simulink model "EulerPIDJoint_Copy"  (Simulink 7.6)
settings: Solver=ode3  StartTime=0.0  StopTime=8  FixedStep=Ts  RelTol=1e-3
InitFcn:
  | eval('Config');
  | eval('RobotCtlCfg');
values from neighbouring files (symbols this model uses):
  a2 = 0    [Config.m]    (also in CtrPlatformCfg.m)
  a3 = 0    [Config.m]    (also in CtrPlatformCfg.m)
  a4 = 0    [Config.m]    (also in CtrPlatformCfg.m)
  a5 = 90    [Config.m]    (also in CtrPlatformCfg.m)
  a6 = 0    [Config.m]    (also in CtrPlatformCfg.m)
  Cen_EU = Cen    [DynEulerTest.m]
  DH_EU = [266     300     0       0       1016     0      174 ... (first row only)    [DynEulerTest.m]
  freq = tvel/radius    (= 1)    [Config.m]    (also in CtrPlatformCfg.m)
  Ft_EU = [0;0;0;0;0;0]    [DynEulerTest.m]
  Gravity = 9.8    [Config.m]    (also in CtrPlatformCfg.m)
  Ie_EU = [Ie1;Ie2;Ie3;Ie4;Ie5;Ie6]    [DynEulerTest.m]
  in1 = [5.2954 -0.2565 -0.6366;-0.2565 4.7000 0.2830;-0.6366 0.2829 5.8635]    [Config.m]    (also in CtrPlatformCfg.m; DynEulerTest.m; EfDynCAD.m = [0.54  -0.01 0.23)
  in2 = [5.8840 0.0072 0.0135;0.0072 6.0178 -0.1907;0.0135 -0.1907 0.3374]    [Config.m]    (also in CtrPlatformCfg.m; DynEulerTest.m; EfDynCAD.m = (R_x*R_z)*in2*(R_x*R_z)')
  in3 = [1.8201 -0.2274 -0.3112;-0.2274 2.2537 -0.1441;-0.3112 -0.1441 1.9485]    [Config.m]    (also in CtrPlatformCfg.m; DynEulerTest.m; EfDynCAD.m = (R_x*R_z)*in3*(R_x*R_z)')
  in4 = [0.0607 -0.0922 0;-0.0922 1.4493 0;0 0 1.4620]    [Config.m]    (also in CtrPlatformCfg.m; DynEulerTest.m = [0.0607 -0.0922 0;-0.0922 1.4493 0;0 0,1.4620]; EfDynCAD.m = (R_y*Rz)*in4*(R_y*Rz)')
  in5 = [0.0191 0.0032 0;0.0032 0.0228 0;0 0 0.0291]    [Config.m]    (also in CtrPlatformCfg.m; DynEulerTest.m; EfDynCAD.m = (R_x*R_y)*in5*(R_x*R_y)')
  in6 = [0.0012 0 0;0 0.0007 0;0 0 0.0007]    [Config.m]    (also in CtrPlatformCfg.m; DynEulerTest.m; EfDynCAD.m = (R_y*Rz)*in6*(R_y*Rz)')
  init_Endx = gd_init(1,4)    [Config.m]    (also in CtrPlatformCfg.m)
  init_Endy = gd_init(2,4)    [Config.m]    (also in CtrPlatformCfg.m)
  init_Endz = gd_init(3,4)    [Config.m]    (also in CtrPlatformCfg.m)
  init_Rot = gd_init(1:3,1:3)    [Config.m]    (also in CtrPlatformCfg.m)
  L = [l1 l2 l3 l4 l5 l6 l7 l8 l9]    [Config.m]    (also in CtrPlatformCfg.m)
  ma1 = 170.31    [Config.m]    (also in CtrPlatformCfg.m; DynEulerTest.m; EfDynCAD.m = 77.75)
  ma2 = 63.74    [Config.m]    (also in CtrPlatformCfg.m; DynEulerTest.m; EfDynCAD.m = 32.31)
  ma3 = 98.98    [Config.m]    (also in CtrPlatformCfg.m; DynEulerTest.m; EfDynCAD.m = 18.61)
  ma4 = 24.46    [Config.m]    (also in CtrPlatformCfg.m; DynEulerTest.m; EfDynCAD.m = 15.65)
  ma5 = 5.24    [Config.m]    (also in CtrPlatformCfg.m; DynEulerTest.m; EfDynCAD.m = 3.32)
  ma6 = 0.6    [Config.m]    (also in CtrPlatformCfg.m; DynEulerTest.m; EfDynCAD.m)
  Ma_EU = Ma    [DynEulerTest.m]
  Rad2Line = Gear*EncRes/(2*pi)    [Config.m]    (also in CtrPlatformCfg.m)
  Ts = 1/FrHz    (= 0.00025)    [Config.m]    (also in CtrPlatformCfg.m)
  tvel = 120    [Config.m]    (also in CtrPlatformCfg.m)
undefined symbols (not defined in the file or in its folder): a1, DiscIntNeverNeededParam, jointAugKp, jointAugKv, PRBSGain, PRBSOffset, PRBSTimeLength, PulseFrq, PulseGain, RobotAxis, SineFrq, SineGain, V2T
libraries: simulink x58, mblibv1 x41, powerlib_extras x7
(part 2 of 5)

== system EulerPIDJoint_Copy/Fanuc/ BodySensor 5 ==
  Avx : Scope
      settings: TimeRange=3  YMin=-150  YMax=125  SaveName=ScopeData62
  Avy : Scope
      settings: TimeRange=3  YMin=-150  YMax=125  SaveName=ScopeData63
  Avz : Scope
      settings: TimeRange=3  YMin=-150  YMax=125  SaveName=ScopeData64
  Awx : Scope
      settings: TimeRange=3  YMin=-150  YMax=125  SaveName=ScopeData65
  Awy : Scope
      settings: TimeRange=3  YMin=-150  YMax=125  SaveName=ScopeData66
  Awz : Scope
      settings: TimeRange=3  YMin=-150  YMax=125  SaveName=ScopeData67
  "Body Sensor " : mblibv1/Sensors &  Actuators/Body Sensor  DialogController=MECH.DynMechDlgSource  SystemSampleTime=-1  UpdateFromCAD=off  PhysicalDomain=Mechanical  PortType=blob  Muxed=on  Pose=off  Angle=on  AngleUnits=deg  ArcVelocity=on  ArcVelocityUnits=deg/s  ArcAcceleration=on  ArcAccelerationUnits=deg/s^2  CoordPosition=off  CoordPositionUnits=mm  Velocity=on  VelocityUnits=mm/s  Acceleration=on  AccelerationUnits=mm/s^2  Quaternion=on  QuaternionDT=off  QuaternionDDT=off  QuaternionUnits=off  OutputVector=[1]  ActiveIO=on  Width=12  DialogClass=MechanicalSensorBlock  ReferenceFrame=Local (Body CS)
  Demux5 : Demux  Outputs=12
  Vx : Scope
      settings: TimeRange=3  YMin=-150  YMax=125  SaveName=ScopeData55
  Vy : Scope
      settings: TimeRange=3  YMin=-150  YMax=125  SaveName=ScopeData57
  Vz : Scope
      settings: TimeRange=3  YMin=-150  YMax=125  SaveName=ScopeData58
  wx : Scope
      settings: TimeRange=3  YMin=-150  YMax=125  SaveName=ScopeData59
  wy : Scope
      settings: TimeRange=3  YMin=-150  YMax=125  SaveName=ScopeData60
  wz : Scope
      settings: TimeRange=3  YMin=-150  YMax=125  SaveName=ScopeData61
  In : PMIOPort  Port=1  Side=Left
  Out : Outport
  wires:
  Demux5/12 -> Awz/1
  Demux5/11 -> Awy/1
  Demux5/10 -> Awx/1
  Demux5/9 -> Avz/1
  Demux5/8 -> Avy/1
  Demux5/7 -> Avx/1
  Demux5/6 -> wz/1
  Demux5/5 -> wy/1
  Demux5/4 -> wx/1
  Demux5/3 -> Vz/1
  Demux5/2 -> Vy/1
  Demux5/1 -> Vx/1
  "Body Sensor "/1 -> Demux5/1, Out/1
  connections:
  In/RConn1 -- "Body Sensor "/LConn1

== system EulerPIDJoint_Copy/Fanuc/ BodySensor 6 ==
  Avx : Scope
      settings: TimeRange=3  YMin=-150  YMax=125  SaveName=ScopeData62
  Avy : Scope
      settings: TimeRange=3  YMin=-150  YMax=125  SaveName=ScopeData63
  Avz : Scope
      settings: TimeRange=3  YMin=-150  YMax=125  SaveName=ScopeData64
  Awx : Scope
      settings: TimeRange=3  YMin=-150  YMax=125  SaveName=ScopeData65
  Awy : Scope
      settings: TimeRange=3  YMin=-150  YMax=125  SaveName=ScopeData66
  Awz : Scope
      settings: TimeRange=3  YMin=-150  YMax=125  SaveName=ScopeData67
  "Body Sensor " : mblibv1/Sensors &  Actuators/Body Sensor  DialogController=MECH.DynMechDlgSource  SystemSampleTime=-1  UpdateFromCAD=off  PhysicalDomain=Mechanical  PortType=blob  Muxed=on  Pose=off  Angle=on  AngleUnits=deg  ArcVelocity=on  ArcVelocityUnits=deg/s  ArcAcceleration=on  ArcAccelerationUnits=deg/s^2  CoordPosition=off  CoordPositionUnits=mm  Velocity=on  VelocityUnits=mm/s  Acceleration=on  AccelerationUnits=mm/s^2  Quaternion=on  QuaternionDT=off  QuaternionDDT=off  QuaternionUnits=off  OutputVector=[1]  ActiveIO=on  Width=12  DialogClass=MechanicalSensorBlock  ReferenceFrame=Local (Body CS)
  Demux5 : Demux  Outputs=12
  Vx : Scope
      settings: TimeRange=3  YMin=-150  YMax=125  SaveName=ScopeData55
  Vy : Scope
      settings: TimeRange=3  YMin=-150  YMax=125  SaveName=ScopeData57
  Vz : Scope
      settings: TimeRange=3  YMin=-150  YMax=125  SaveName=ScopeData58
  wx : Scope
      settings: TimeRange=3  YMin=-150  YMax=125  SaveName=ScopeData59
  wy : Scope
      settings: TimeRange=3  YMin=-150  YMax=125  SaveName=ScopeData60
  wz : Scope
      settings: TimeRange=3  YMin=-150  YMax=125  SaveName=ScopeData61
  In : PMIOPort  Port=1  Side=Left
  Out : Outport
  wires:
  "Body Sensor "/1 -> Out/1, Demux5/1
  Demux5/1 -> Vx/1
  Demux5/2 -> Vy/1
  Demux5/3 -> Vz/1
  Demux5/4 -> wx/1
  Demux5/5 -> wy/1
  Demux5/6 -> wz/1
  Demux5/7 -> Avx/1
  Demux5/8 -> Avy/1
  Demux5/9 -> Avz/1
  Demux5/10 -> Awx/1
  Demux5/11 -> Awy/1
  Demux5/12 -> Awz/1
  connections:
  In/RConn1 -- "Body Sensor "/LConn1

== system EulerPIDJoint_Copy/Fanuc/ EndSensor ==
  Avx : Scope
      settings: TimeRange=3  YMin=-150  YMax=125  SaveName=ScopeData62
  Avy : Scope
      settings: TimeRange=3  YMin=-150  YMax=125  SaveName=ScopeData63
  Avz : Scope
      settings: TimeRange=3  YMin=-150  YMax=125  SaveName=ScopeData64
  Awx : Scope
      settings: TimeRange=3  YMin=-150  YMax=125  SaveName=ScopeData65
  Awy : Scope
      settings: TimeRange=3  YMin=-150  YMax=125  SaveName=ScopeData66
  Awz : Scope
      settings: TimeRange=3  YMin=-150  YMax=125  SaveName=ScopeData67
  "Body Sensor " : mblibv1/Sensors &  Actuators/Body Sensor  DialogController=MECH.DynMechDlgSource  SystemSampleTime=-1  UpdateFromCAD=off  PhysicalDomain=Mechanical  PortType=blob  Muxed=on  Pose=off  Angle=on  AngleUnits=deg  ArcVelocity=on  ArcVelocityUnits=deg/s  ArcAcceleration=on  ArcAccelerationUnits=deg/s^2  CoordPosition=on  CoordPositionUnits=mm  Velocity=on  VelocityUnits=mm/s  Acceleration=on  AccelerationUnits=mm/s^2  Quaternion=on  QuaternionDT=off  QuaternionDDT=off  QuaternionUnits=off  OutputVector=[1]  ActiveIO=on  Width=15  DialogClass=MechanicalSensorBlock  ReferenceFrame=Absolute (World)
  Demux5 : Demux  Outputs=15
  EndX : ToWorkspace  VariableName=EndX  SampleTime=-1  SaveFormat=Structure
  EndY : ToWorkspace  VariableName=EndY  SampleTime=-1  SaveFormat=Structure
  EndZ : ToWorkspace  VariableName=EndZ  SampleTime=-1  SaveFormat=Structure
  Vx : Scope
      settings: TimeRange=3  YMin=-150  YMax=125  SaveName=ScopeData55
  Vy : Scope
      settings: TimeRange=3  YMin=-150  YMax=125  SaveName=ScopeData57
  Vz : Scope
      settings: TimeRange=3  YMin=-150  YMax=125  SaveName=ScopeData58
  X : Scope
      settings: TimeRange=3  YMin=-150  YMax=125  SaveName=ScopeData36
  Y : Scope
      settings: TimeRange=3  YMin=-150  YMax=125  SaveName=ScopeData37
  Z : Scope
      settings: TimeRange=3  YMin=-150  YMax=125  SaveName=ScopeData38
  wx : Scope
      settings: TimeRange=3  YMin=-150  YMax=125  SaveName=ScopeData59
  wy : Scope
      settings: TimeRange=3  YMin=-150  YMax=125  SaveName=ScopeData60
  wz : Scope
      settings: TimeRange=3  YMin=-150  YMax=125  SaveName=ScopeData61
  In : PMIOPort  Port=1  Side=Left
  Out : Outport
  wires:
  "Body Sensor "/1 -> Demux5/1, Out/1
  Demux5/4 -> Vx/1
  Demux5/5 -> Vy/1
  Demux5/6 -> Vz/1
  Demux5/7 -> wx/1
  Demux5/8 -> wy/1
  Demux5/9 -> wz/1
  Demux5/10 -> Avx/1
  Demux5/11 -> Avy/1
  Demux5/12 -> Avz/1
  Demux5/13 -> Awx/1
  Demux5/14 -> Awy/1
  Demux5/15 -> Awz/1
  Demux5/1 -> EndX/1, X/1
  Demux5/2 -> EndY/1, Y/1
  Demux5/3 -> EndZ/1, Z/1
  connections:
  In/RConn1 -- "Body Sensor "/LConn1

== system EulerPIDJoint_Copy/Fanuc/JointSensor1 ==
  Angle Acceleration : Scope
      settings: SaveName=ScopeData32
  Angle Velocity : Scope
      settings: SaveName=ScopeData31
  Anlge : Scope
      settings: SaveName=ScopeData30
  Computed Torque : Scope
      settings: SaveName=ScopeData33
  Demux : Demux  Outputs=10
  Reaction Force : Scope  NumInputPorts=3
      settings: YMin=-5~-5~-5  YMax=5~5~5  SaveName=ScopeData12
  Reaction Torque : Scope  NumInputPorts=3
      settings: YMin=-5~-5~-5  YMax=5~5~5  SaveName=ScopeData34
  Sensor1 : mblibv1/Sensors &  Actuators/Joint Sensor  DialogController=MECH.DynMechDlgSource  SystemSampleTime=-1  UpdateFromCAD=off  PhysicalDomain=Mechanical  PortType=blob  Muxed=on  Pose=off  Angle=on  AngleUnits=deg  ArcVelocity=on  ArcVelocityUnits=deg/s  ArcAcceleration=on  ArcAccelerationUnits=deg/s^2  CoordPosition=on  CoordPositionUnits=m  Velocity=off  VelocityUnits=m/s  Acceleration=off  AccelerationUnits=m/s^2  Quaternion=on  QuaternionDT=off  QuaternionDDT=off  QuaternionUnits=off  OutputVector=[1]  ActiveIO=on  Width=10  DialogClass=MechanicalSensorBlock  Primitive=R1  Force=off  ForceUnits=N  Torque=on  TorqueUnits=N*m  ReferenceFrame=Absolute (World)  ReactionSensedSide=Follower  ReactionReferenceFrame=Absolute (World)  ReactionForce=on  ReactionForceUnits=N  ReactionMoment=on  ReactionMomentUnits=N*m
  In : PMIOPort  Port=1  Side=Left
  Out : Outport
  wires:
  Sensor1/1 -> Demux/1, Out/1
  Demux/2 -> Angle Velocity/1
  Demux/1 -> Anlge/1
  Demux/3 -> Angle Acceleration/1
  Demux/4 -> Computed Torque/1
  Demux/5 -> Reaction Torque/1
  Demux/6 -> Reaction Torque/2
  Demux/7 -> Reaction Torque/3
  Demux/8 -> Reaction Force/1
  Demux/9 -> Reaction Force/2
  Demux/10 -> Reaction Force/3
  connections:
  In/RConn1 -- Sensor1/LConn1

== system EulerPIDJoint_Copy/Fanuc/JointSensor2 ==
  Angle Acceleration : Scope
      settings: SaveName=ScopeData32
  Angle Velocity : Scope
      settings: SaveName=ScopeData31
  Anlge : Scope
      settings: SaveName=ScopeData30
  Computed Torque : Scope
      settings: SaveName=ScopeData33
  Demux : Demux  Outputs=10
  Reaction Force : Scope  NumInputPorts=3
      settings: YMin=-5~-5~-5  YMax=5~5~5  SaveName=ScopeData12
  Reaction Torque : Scope  NumInputPorts=3
      settings: YMin=-5~-5~-5  YMax=5~5~5  SaveName=ScopeData34
  Sensor1 : mblibv1/Sensors &  Actuators/Joint Sensor  DialogController=MECH.DynMechDlgSource  SystemSampleTime=-1  UpdateFromCAD=off  PhysicalDomain=Mechanical  PortType=blob  Muxed=on  Pose=off  Angle=on  AngleUnits=deg  ArcVelocity=on  ArcVelocityUnits=deg/s  ArcAcceleration=on  ArcAccelerationUnits=deg/s^2  CoordPosition=on  CoordPositionUnits=m  Velocity=off  VelocityUnits=m/s  Acceleration=off  AccelerationUnits=m/s^2  Quaternion=on  QuaternionDT=off  QuaternionDDT=off  QuaternionUnits=off  OutputVector=[1]  ActiveIO=on  Width=10  DialogClass=MechanicalSensorBlock  Primitive=R1  Force=off  ForceUnits=N  Torque=on  TorqueUnits=N*m  ReferenceFrame=Absolute (World)  ReactionSensedSide=Follower  ReactionReferenceFrame=Absolute (World)  ReactionForce=on  ReactionForceUnits=N  ReactionMoment=on  ReactionMomentUnits=N*m
  In : PMIOPort  Port=1  Side=Left
  Out : Outport
  wires:
  Demux/10 -> Reaction Force/3
  Demux/9 -> Reaction Force/2
  Demux/8 -> Reaction Force/1
  Demux/7 -> Reaction Torque/3
  Demux/6 -> Reaction Torque/2
  Demux/5 -> Reaction Torque/1
  Demux/4 -> Computed Torque/1
  Demux/3 -> Angle Acceleration/1
  Demux/1 -> Anlge/1
  Demux/2 -> Angle Velocity/1
  Sensor1/1 -> Out/1, Demux/1
  connections:
  In/RConn1 -- Sensor1/LConn1

== system EulerPIDJoint_Copy/Fanuc/JointSensor3 ==
  Angle Acceleration : Scope
      settings: SaveName=ScopeData32
  Angle Velocity : Scope
      settings: SaveName=ScopeData31
  Anlge : Scope
      settings: SaveName=ScopeData30
  Computed Torque : Scope
      settings: SaveName=ScopeData33
  Demux : Demux  Outputs=10
  Reaction Force : Scope  NumInputPorts=3
      settings: YMin=-5~-5~-5  YMax=5~5~5  SaveName=ScopeData12
  Reaction Torque : Scope  NumInputPorts=3
      settings: YMin=-5~-5~-5  YMax=5~5~5  SaveName=ScopeData34
  Sensor1 : mblibv1/Sensors &  Actuators/Joint Sensor  DialogController=MECH.DynMechDlgSource  SystemSampleTime=-1  UpdateFromCAD=off  PhysicalDomain=Mechanical  PortType=blob  Muxed=on  Pose=off  Angle=on  AngleUnits=deg  ArcVelocity=on  ArcVelocityUnits=deg/s  ArcAcceleration=on  ArcAccelerationUnits=deg/s^2  CoordPosition=on  CoordPositionUnits=m  Velocity=off  VelocityUnits=m/s  Acceleration=off  AccelerationUnits=m/s^2  Quaternion=on  QuaternionDT=off  QuaternionDDT=off  QuaternionUnits=off  OutputVector=[1]  ActiveIO=on  Width=10  DialogClass=MechanicalSensorBlock  Primitive=R1  Force=off  ForceUnits=N  Torque=on  TorqueUnits=N*m  ReferenceFrame=Absolute (World)  ReactionSensedSide=Follower  ReactionReferenceFrame=Absolute (World)  ReactionForce=on  ReactionForceUnits=N  ReactionMoment=on  ReactionMomentUnits=N*m
  In : PMIOPort  Port=1  Side=Left
  Out : Outport
  wires:
  Sensor1/1 -> Demux/1, Out/1
  Demux/2 -> Angle Velocity/1
  Demux/1 -> Anlge/1
  Demux/3 -> Angle Acceleration/1
  Demux/4 -> Computed Torque/1
  Demux/5 -> Reaction Torque/1
  Demux/6 -> Reaction Torque/2
  Demux/7 -> Reaction Torque/3
  Demux/8 -> Reaction Force/1
  Demux/9 -> Reaction Force/2
  Demux/10 -> Reaction Force/3
  connections:
  In/RConn1 -- Sensor1/LConn1

== system EulerPIDJoint_Copy/Fanuc/JointSensor4 ==
  Angle Acceleration : Scope
      settings: SaveName=ScopeData32
  Angle Velocity : Scope
      settings: SaveName=ScopeData31
  Anlge : Scope
      settings: SaveName=ScopeData30
  Computed Torque : Scope
      settings: SaveName=ScopeData33
  Demux : Demux  Outputs=10
  Reaction Force : Scope  NumInputPorts=3
      settings: YMin=-5~-5~-5  YMax=5~5~5  SaveName=ScopeData12
  Reaction Torque : Scope  NumInputPorts=3
      settings: YMin=-5~-5~-5  YMax=5~5~5  SaveName=ScopeData34
  Sensor1 : mblibv1/Sensors &  Actuators/Joint Sensor  DialogController=MECH.DynMechDlgSource  SystemSampleTime=-1  UpdateFromCAD=off  PhysicalDomain=Mechanical  PortType=blob  Muxed=on  Pose=off  Angle=on  AngleUnits=deg  ArcVelocity=on  ArcVelocityUnits=deg/s  ArcAcceleration=on  ArcAccelerationUnits=deg/s^2  CoordPosition=on  CoordPositionUnits=m  Velocity=off  VelocityUnits=m/s  Acceleration=off  AccelerationUnits=m/s^2  Quaternion=on  QuaternionDT=off  QuaternionDDT=off  QuaternionUnits=off  OutputVector=[1]  ActiveIO=on  Width=10  DialogClass=MechanicalSensorBlock  Primitive=R1  Force=off  ForceUnits=N  Torque=on  TorqueUnits=N*m  ReferenceFrame=Absolute (World)  ReactionSensedSide=Follower  ReactionReferenceFrame=Absolute (World)  ReactionForce=on  ReactionForceUnits=N  ReactionMoment=on  ReactionMomentUnits=N*m
  In : PMIOPort  Port=1  Side=Left
  Out : Outport
  wires:
  Demux/10 -> Reaction Force/3
  Demux/9 -> Reaction Force/2
  Demux/8 -> Reaction Force/1
  Demux/7 -> Reaction Torque/3
  Demux/6 -> Reaction Torque/2
  Demux/5 -> Reaction Torque/1
  Demux/4 -> Computed Torque/1
  Demux/3 -> Angle Acceleration/1
  Demux/1 -> Anlge/1
  Demux/2 -> Angle Velocity/1
  Sensor1/1 -> Out/1, Demux/1
  connections:
  In/RConn1 -- Sensor1/LConn1

== system EulerPIDJoint_Copy/Fanuc/JointSensor5 ==
  Angle Acceleration : Scope
      settings: SaveName=ScopeData32
  Angle Velocity : Scope
      settings: SaveName=ScopeData31
  Anlge : Scope
      settings: SaveName=ScopeData30
  Computed Torque : Scope
      settings: SaveName=ScopeData33
  Demux : Demux  Outputs=10
  Reaction Force : Scope  NumInputPorts=3
      settings: YMin=-5~-5~-5  YMax=5~5~5  SaveName=ScopeData12
  Reaction Torque : Scope  NumInputPorts=3
      settings: YMin=-5~-5~-5  YMax=5~5~5  SaveName=ScopeData34
  Sensor1 : mblibv1/Sensors &  Actuators/Joint Sensor  DialogController=MECH.DynMechDlgSource  SystemSampleTime=-1  UpdateFromCAD=off  PhysicalDomain=Mechanical  PortType=blob  Muxed=on  Pose=off  Angle=on  AngleUnits=deg  ArcVelocity=on  ArcVelocityUnits=deg/s  ArcAcceleration=on  ArcAccelerationUnits=deg/s^2  CoordPosition=on  CoordPositionUnits=m  Velocity=off  VelocityUnits=m/s  Acceleration=off  AccelerationUnits=m/s^2  Quaternion=on  QuaternionDT=off  QuaternionDDT=off  QuaternionUnits=off  OutputVector=[1]  ActiveIO=on  Width=10  DialogClass=MechanicalSensorBlock  Primitive=R1  Force=off  ForceUnits=N  Torque=on  TorqueUnits=N*m  ReferenceFrame=Absolute (World)  ReactionSensedSide=Follower  ReactionReferenceFrame=Absolute (World)  ReactionForce=on  ReactionForceUnits=N  ReactionMoment=on  ReactionMomentUnits=N*m
  In : PMIOPort  Port=1  Side=Left
  Out : Outport
  wires:
  Sensor1/1 -> Demux/1, Out/1
  Demux/2 -> Angle Velocity/1
  Demux/1 -> Anlge/1
  Demux/3 -> Angle Acceleration/1
  Demux/4 -> Computed Torque/1
  Demux/5 -> Reaction Torque/1
  Demux/6 -> Reaction Torque/2
  Demux/7 -> Reaction Torque/3
  Demux/8 -> Reaction Force/1
  Demux/9 -> Reaction Force/2
  Demux/10 -> Reaction Force/3
  connections:
  In/RConn1 -- Sensor1/LConn1

== system EulerPIDJoint_Copy/Fanuc/JointSensor6 ==
  Angle Acceleration : Scope
      settings: SaveName=ScopeData32
  Angle Velocity : Scope
      settings: SaveName=ScopeData31
  Anlge : Scope
      settings: SaveName=ScopeData30
  Computed Torque : Scope
      settings: SaveName=ScopeData33
  Demux : Demux  Outputs=10
  Reaction Force : Scope  NumInputPorts=3
      settings: YMin=-5~-5~-5  YMax=5~5~5  SaveName=ScopeData12
  Reaction Torque : Scope  NumInputPorts=3
      settings: YMin=-5~-5~-5  YMax=5~5~5  SaveName=ScopeData34
  Sensor1 : mblibv1/Sensors &  Actuators/Joint Sensor  DialogController=MECH.DynMechDlgSource  SystemSampleTime=-1  UpdateFromCAD=off  PhysicalDomain=Mechanical  PortType=blob  Muxed=on  Pose=off  Angle=on  AngleUnits=deg  ArcVelocity=on  ArcVelocityUnits=deg/s  ArcAcceleration=on  ArcAccelerationUnits=deg/s^2  CoordPosition=on  CoordPositionUnits=m  Velocity=off  VelocityUnits=m/s  Acceleration=off  AccelerationUnits=m/s^2  Quaternion=on  QuaternionDT=off  QuaternionDDT=off  QuaternionUnits=off  OutputVector=[1]  ActiveIO=on  Width=10  DialogClass=MechanicalSensorBlock  Primitive=R1  Force=off  ForceUnits=N  Torque=on  TorqueUnits=N*m  ReferenceFrame=Absolute (World)  ReactionSensedSide=Follower  ReactionReferenceFrame=Absolute (World)  ReactionForce=on  ReactionForceUnits=N  ReactionMoment=on  ReactionMomentUnits=N*m
  In : PMIOPort  Port=1  Side=Left
  Out : Outport
  wires:
  Demux/10 -> Reaction Force/3
  Demux/9 -> Reaction Force/2
  Demux/8 -> Reaction Force/1
  Demux/7 -> Reaction Torque/3
  Demux/6 -> Reaction Torque/2
  Demux/5 -> Reaction Torque/1
  Demux/4 -> Computed Torque/1
  Demux/3 -> Angle Acceleration/1
  Demux/1 -> Anlge/1
  Demux/2 -> Angle Velocity/1
  Sensor1/1 -> Out/1, Demux/1
  connections:
  In/RConn1 -- Sensor1/LConn1

== system EulerPIDJoint_Copy/Signal Re-group/Re-group ==
  JntVelAcc_R1 : Inport
  Torque_R1 : Inport  Port=2
  GeneralForce_R1 : Inport  Port=3
  JntVelAcc_R2 : Inport  Port=4
  Torque_R2 : Inport  Port=5
  GeneralForce_R2 : Inport  Port=6
  JntVelAcc_R3 : Inport  Port=7
  Torque_R3 : Inport  Port=8
  GeneralForce_R3 : Inport  Port=9
  JntVelAcc_R4 : Inport  Port=10
  Torque_R4 : Inport  Port=11
  GeneralForce_R4 : Inport  Port=12
  JntVelAcc_R5 : Inport  Port=13
  Torque_R5 : Inport  Port=14
  GeneralForce_R5 : Inport  Port=15
  JntVelAcc_R6 : Inport  Port=16
  Torque_R6 : Inport  Port=17
  GeneralForce_R6 : Inport  Port=18
  Mux : Mux  Inputs=6
  Mux1 : Mux  Inputs=6
  Mux2 : Mux  Inputs=6
  JntVelAcc : Outport
  Torque : Outport  Port=2
  GeneralForce : Outport  Port=3
  wires:
  JntVelAcc_R1/1 -> Mux/1
  JntVelAcc_R2/1 -> Mux/2
  JntVelAcc_R3/1 -> Mux/3
  JntVelAcc_R4/1 -> Mux/4
  JntVelAcc_R5/1 -> Mux/5
  JntVelAcc_R6/1 -> Mux/6
  Torque_R1/1 -> Mux1/1
  Torque_R2/1 -> Mux1/2
  Torque_R3/1 -> Mux1/3
  Torque_R4/1 -> Mux1/4
  Torque_R5/1 -> Mux1/5
  Torque_R6/1 -> Mux1/6
  GeneralForce_R1/1 -> Mux2/1
  GeneralForce_R2/1 -> Mux2/2
  GeneralForce_R3/1 -> Mux2/3
  GeneralForce_R4/1 -> Mux2/4
  GeneralForce_R5/1 -> Mux2/5
  GeneralForce_R6/1 -> Mux2/6
  Mux/1 -> JntVelAcc/1
  Mux1/1 -> Torque/1
  Mux2/1 -> GeneralForce/1

== system EulerPIDJoint_Copy/Signal Re-group/Re-group JntVelAcc ==
  JntVelAcc : Inport
  Demux2 : Demux  Outputs=18
  Mux : Mux  Inputs=6
  Mux1 : Mux  Inputs=6
  Mux2 : Mux  Inputs=6
  Mux3 : Mux  Inputs=3
  ReJntVelAcc : Outport
  wires:
  JntVelAcc/1 -> Demux2/1
  Demux2/1 -> Mux/1
  Demux2/2 -> Mux1/1
  Demux2/3 -> Mux2/1
  Demux2/4 -> Mux/2
  Demux2/5 -> Mux1/2
  Demux2/6 -> Mux2/2
  Demux2/7 -> Mux/3
  Demux2/8 -> Mux1/3
  Demux2/9 -> Mux2/3
  Demux2/10 -> Mux/4
  Demux2/11 -> Mux1/4
  Demux2/12 -> Mux2/4
  Demux2/13 -> Mux/5
  Demux2/14 -> Mux1/5
  Demux2/15 -> Mux2/5
  Demux2/16 -> Mux/6
  Demux2/17 -> Mux1/6
  Demux2/18 -> Mux2/6
  Mux/1 -> Mux3/1
  Mux1/1 -> Mux3/2
  Mux2/1 -> Mux3/3
  Mux3/1 -> ReJntVelAcc/1

== system EulerPIDJoint_Copy/Signal Re-group/Re-group_B ==
  In_B1 : Inport
  In_B2 : Inport  Port=2
  In_B3 : Inport  Port=3
  In_B4 : Inport  Port=4
  In_B5 : Inport  Port=5
  In_B6 : Inport  Port=6
  Demux{1..6} (6 alike) : Demux  Outputs=2
  Mux : Mux  Inputs=6
  Mux1 : Mux  Inputs=6
  GeneralVel : Outport
  GeneralAcc : Outport  Port=2
  wires:
  In_B1/1 -> Demux2/1
  In_B2/1 -> Demux1/1
  In_B3/1 -> Demux3/1
  In_B4/1 -> Demux4/1
  In_B5/1 -> Demux5/1
  In_B6/1 -> Demux6/1
  Demux2/1 -> Mux/1
  Demux1/1 -> Mux/2
  Demux3/1 -> Mux/3
  Demux4/1 -> Mux/4
  Demux5/1 -> Mux/5
  Demux6/1 -> Mux/6
  Demux2/2 -> Mux1/1
  Demux1/2 -> Mux1/2
  Demux3/2 -> Mux1/3
  Demux4/2 -> Mux1/4
  Demux5/2 -> Mux1/5
  Demux6/2 -> Mux1/6
  Mux1/1 -> GeneralAcc/1
  Mux/1 -> GeneralVel/1

== system EulerPIDJoint_Copy/Signal Re-group/Re-group_R1 ==
  In_R1 : Inport
  Demux2 : Demux  Outputs=10
  Mux : Mux  Inputs=3
  Mux1 : Mux  Inputs=3
  Mux2 : Mux  Inputs=3
  Mux3 : Mux  Inputs=2
  JntVelAcc_R1 : Outport
  Torque_R1 : Outport  Port=2
  GeneralForce_R1 : Outport  Port=3
  wires:
  In_R1/1 -> Demux2/1
  Demux2/1 -> Mux/1
  Demux2/2 -> Mux/2
  Demux2/3 -> Mux/3
  Demux2/4 -> Torque_R1/1
  Demux2/5 -> Mux1/1
  Demux2/6 -> Mux1/2
  Demux2/7 -> Mux1/3
  Demux2/8 -> Mux2/1
  Demux2/9 -> Mux2/2
  Demux2/10 -> Mux2/3
  Mux1/1 -> Mux3/2
  Mux2/1 -> Mux3/1
  Mux/1 -> JntVelAcc_R1/1
  Mux3/1 -> GeneralForce_R1/1

== system EulerPIDJoint_Copy/Signal Re-group/Re-group_R2 ==
  In_R2 : Inport
  Demux2 : Demux  Outputs=10
  Mux : Mux  Inputs=3
  Mux1 : Mux  Inputs=3
  Mux2 : Mux  Inputs=3
  Mux3 : Mux  Inputs=2
  JntVelAcc_R2 : Outport
  Torque_R2 : Outport  Port=2
  GeneralForce_R2 : Outport  Port=3
  wires:
  Mux3/1 -> GeneralForce_R2/1
  Mux/1 -> JntVelAcc_R2/1
  Mux2/1 -> Mux3/1
  Mux1/1 -> Mux3/2
  Demux2/10 -> Mux2/3
  Demux2/9 -> Mux2/2
  Demux2/8 -> Mux2/1
  Demux2/7 -> Mux1/3
  Demux2/6 -> Mux1/2
  Demux2/5 -> Mux1/1
  Demux2/4 -> Torque_R2/1
  Demux2/3 -> Mux/3
  Demux2/2 -> Mux/2
  Demux2/1 -> Mux/1
  In_R2/1 -> Demux2/1

== system EulerPIDJoint_Copy/Signal Re-group/Re-group_R3 ==
  In_R3 : Inport
  Demux2 : Demux  Outputs=10
  Mux : Mux  Inputs=3
  Mux1 : Mux  Inputs=3
  Mux2 : Mux  Inputs=3
  Mux3 : Mux  Inputs=2
  JntVelAcc_R3 : Outport
  Torque_R3 : Outport  Port=2
  GeneralForce_R3 : Outport  Port=3
  wires:
  In_R3/1 -> Demux2/1
  Demux2/1 -> Mux/1
  Demux2/2 -> Mux/2
  Demux2/3 -> Mux/3
  Demux2/4 -> Torque_R3/1
  Demux2/5 -> Mux1/1
  Demux2/6 -> Mux1/2
  Demux2/7 -> Mux1/3
  Demux2/8 -> Mux2/1
  Demux2/9 -> Mux2/2
  Demux2/10 -> Mux2/3
  Mux1/1 -> Mux3/2
  Mux2/1 -> Mux3/1
  Mux/1 -> JntVelAcc_R3/1
  Mux3/1 -> GeneralForce_R3/1

== system EulerPIDJoint_Copy/Signal Re-group/Re-group_R4 ==
  In_R4 : Inport
  Demux2 : Demux  Outputs=10
  Mux : Mux  Inputs=3
  Mux1 : Mux  Inputs=3
  Mux2 : Mux  Inputs=3
  Mux3 : Mux  Inputs=2
  JntVelAcc_R4 : Outport
  Torque_R4 : Outport  Port=2
  GeneralForce_R4 : Outport  Port=3
  wires:
  Mux3/1 -> GeneralForce_R4/1
  Mux/1 -> JntVelAcc_R4/1
  Mux2/1 -> Mux3/1
  Mux1/1 -> Mux3/2
  Demux2/10 -> Mux2/3
  Demux2/9 -> Mux2/2
  Demux2/8 -> Mux2/1
  Demux2/7 -> Mux1/3
  Demux2/6 -> Mux1/2
  Demux2/5 -> Mux1/1
  Demux2/4 -> Torque_R4/1
  Demux2/3 -> Mux/3
  Demux2/2 -> Mux/2
  Demux2/1 -> Mux/1
  In_R4/1 -> Demux2/1

== system EulerPIDJoint_Copy/Signal Re-group/Re-group_R5 ==
  In_R5 : Inport
  Demux2 : Demux  Outputs=10
  Mux : Mux  Inputs=3
  Mux1 : Mux  Inputs=3
  Mux2 : Mux  Inputs=3
  Mux3 : Mux  Inputs=2
  JntVelAcc_R5 : Outport
  Torque_R5 : Outport  Port=2
  GeneralForce_R5 : Outport  Port=3
  wires:
  In_R5/1 -> Demux2/1
  Demux2/1 -> Mux/1
  Demux2/2 -> Mux/2
  Demux2/3 -> Mux/3
  Demux2/4 -> Torque_R5/1
  Demux2/5 -> Mux1/1
  Demux2/6 -> Mux1/2
  Demux2/7 -> Mux1/3
  Demux2/8 -> Mux2/1
  Demux2/9 -> Mux2/2
  Demux2/10 -> Mux2/3
  Mux1/1 -> Mux3/2
  Mux2/1 -> Mux3/1
  Mux/1 -> JntVelAcc_R5/1
  Mux3/1 -> GeneralForce_R5/1

== system EulerPIDJoint_Copy/Signal Re-group/Re-group_R6 ==
  In_R6 : Inport
  Demux2 : Demux  Outputs=10
  Mux : Mux  Inputs=3
  Mux1 : Mux  Inputs=3
  Mux2 : Mux  Inputs=3
  Mux3 : Mux  Inputs=2
  JntVelAcc_R6 : Outport
  Torque_R6 : Outport  Port=2
  GeneralForce_R6 : Outport  Port=3
  wires:
  Mux3/1 -> GeneralForce_R6/1
  Mux/1 -> JntVelAcc_R6/1
  Mux2/1 -> Mux3/1
  Mux1/1 -> Mux3/2
  Demux2/10 -> Mux2/3
  Demux2/9 -> Mux2/2
  Demux2/8 -> Mux2/1
  Demux2/7 -> Mux1/3
  Demux2/6 -> Mux1/2
  Demux2/5 -> Mux1/1
  Demux2/4 -> Torque_R6/1
  Demux2/3 -> Mux/3
  Demux2/2 -> Mux/2
  Demux2/1 -> Mux/1
  In_R6/1 -> Demux2/1

== system EulerPIDJoint_Copy/Trajectory Generator/Circle in Descartes Space ==
  Difference{,1..3} (4 alike) : simulink/Discrete/Difference  SystemSampleTime=-1  ICPrevInput=0.0  OutMin=[]  OutMax=[]  OutDataType=fixdt(1, 16)  OutScaling=2^-10  DoSatur=off
  Discrete-Time Integrator : DiscreteIntegrator  InitialCondition=init_Endx  SampleTime=Ts  ICPrevOutput=DiscIntNeverNeededParam  ICPrevScaledInput=DiscIntNeverNeededParam
  Discrete-Time Integrator1 : DiscreteIntegrator  InitialCondition=init_Endy  SampleTime=Ts  ICPrevOutput=DiscIntNeverNeededParam  ICPrevScaledInput=DiscIntNeverNeededParam
  Discrete-Time Integrator2 : DiscreteIntegrator  InitialCondition=init_Endz  SampleTime=Ts  ICPrevOutput=DiscIntNeverNeededParam  ICPrevScaledInput=DiscIntNeverNeededParam
  EndVelocity : Subsystem
  Inverse Kinematic : Stateflow chart  TreatAsAtomicUnit=on
  Jacobian : Stateflow chart  TreatAsAtomicUnit=on
  Mux{1..3,5..6} (5 alike) : Mux  Inputs=3
  Mux4 : Mux  Inputs=5
  Rad2Deg : Gain  Gain=180/pi
  "Re-group " : Subsystem
  Zero : Gain  Gain=0
  Zero1 : Gain  Gain=1/Ts
  Zero2 : Gain  Gain=1/Ts
  Ref_JJVVAA : Outport
  RefEnd : Outport  Port=2
  Ref_JVAJVA : Outport  Port=3
  wires:
  Discrete-Time Integrator/1 -> Mux2/1
  Discrete-Time Integrator1/1 -> Mux2/2
  EndVelocity/1(EndVx) -> Mux1/1, Mux5/1, Difference/1, Discrete-Time Integrator/1
  EndVelocity/2(EndVy) -> Mux1/2, Mux5/2, Difference1/1, Discrete-Time Integrator1/1
  EndVelocity/3(EndVz) -> Mux1/3, Mux5/3, Difference2/1, Discrete-Time Integrator2/1
  Discrete-Time Integrator2/1 -> Mux2/3
  Mux2/1 -> Inverse Kinematic/1(EndPos), Mux4/1
  Inverse Kinematic/1(Theta) -> Jacobian/1(Theta), Mux3/1
  Mux4/1 -> RefEnd/1
  Difference/1 -> Mux6/1
  Difference1/1 -> Mux6/2
  Difference2/1 -> Mux6/3
  Mux1/1 -> Jacobian/2(EndVel)
  Jacobian/1(Omega) -> Mux3/2, Difference3/1
  Difference3/1 -> Zero2/1
  Mux3/1 -> Ref_JJVVAA/1, "Re-group "/1(JJVVAA)
  "Re-group "/1(JVAJVA) -> Rad2Deg/1
  Mux5/1 -> Mux4/2
  Mux6/1 -> Zero1/1
  Zero/1 -> Mux4/3, Mux4/5
  Rad2Deg/1 -> Ref_JVAJVA/1
  Zero1/1 -> Mux4/4, Zero/1
  Zero2/1 -> Mux3/3

== system EulerPIDJoint_Copy/Trajectory Generator/Line in Joint Space ==
  Derivative{1..6,8} (7 alike) : Derivative
  EndAngule : Subsystem
  Forward : Stateflow chart  TreatAsAtomicUnit=on
  Integrator : Integrator  InitialCondition=a1/180*pi
  Integrator1 : Integrator  InitialCondition=a2/180*pi
  Integrator2 : Integrator  InitialCondition=a3/180*pi
  Integrator3 : Integrator  InitialCondition=a4/180*pi
  Integrator4 : Integrator  InitialCondition=a5/180*pi
  Integrator5 : Integrator  InitialCondition=a6/180*pi
  Jacobian : Stateflow chart  TreatAsAtomicUnit=on
  Mux1 : Mux  Inputs=6
  Mux2 : Mux  Inputs=6
  Mux3 : Mux  Inputs=3
  Mux4 : Mux  Inputs=6
  Mux5 : Mux  Inputs=5
  Rad2Deg : Gain  Gain=180/pi
  "Re-group " : Subsystem
  Zero : Gain  Gain=0
  Ref_JJVVAA : Outport
  RefEnd : Outport  Port=2
  Ref_JVAJVA : Outport  Port=3
  wires:
  Forward/1(EndPos) -> Mux5/1, Zero/1
  Mux5/1 -> RefEnd/1
  Mux4/1 -> Mux3/3
  Mux1/1 -> Jacobian/1(Theta), Mux3/1, Forward/1(Theta)
  Mux2/1 -> Jacobian/2(Omega), Mux3/2
  Derivative6/1 -> Mux4/6
  Derivative5/1 -> Mux4/5
  Derivative4/1 -> Mux4/4
  Derivative2/1 -> Mux4/3
  Derivative1/1 -> Mux4/2
  Derivative3/1 -> Mux4/1
  Integrator5/1 -> Mux1/6
  Integrator4/1 -> Mux1/5
  Integrator3/1 -> Mux1/4
  Integrator2/1 -> Mux1/3
  Integrator1/1 -> Mux1/2
  Integrator/1 -> Mux1/1
  EndAngule/6(Omega6) -> Derivative6/1, Mux2/6, Integrator5/1
  EndAngule/5(Omega5) -> Derivative5/1, Mux2/5, Integrator4/1
  EndAngule/4(Omega4) -> Derivative4/1, Mux2/4, Integrator3/1
  EndAngule/3(Omega3) -> Derivative2/1, Mux2/3, Integrator2/1
  EndAngule/2(Omega2) -> Derivative1/1, Mux2/2, Integrator1/1
  EndAngule/1(Omega1) -> Derivative3/1, Mux2/1, Integrator/1
  Mux3/1 -> Ref_JJVVAA/1, "Re-group "/1(JJVVAA)
  "Re-group "/1(JVAJVA) -> Rad2Deg/1
  Jacobian/1(EndVel) -> Derivative8/1, Mux5/2
  Derivative8/1 -> Mux5/4
  Zero/1 -> Mux5/3, Mux5/5
  Rad2Deg/1 -> Ref_JVAJVA/1

== system EulerPIDJoint_Copy/Trajectory Generator/Still ==
  Derivative : Derivative
  Derivative1 : Derivative
  Derivative3 : Derivative
  Drivative2 : Derivative
  EndVelocity : Subsystem
  Integrator : Integrator  InitialCondition=init_Endx
  Integrator1 : Integrator  InitialCondition=init_Endy
  Integrator2 : Integrator  InitialCondition=init_Endz
  Inverse Kinematic : Stateflow chart  TreatAsAtomicUnit=on
  Jacobian : Stateflow chart  TreatAsAtomicUnit=on
  Mux{1..3,5..6} (5 alike) : Mux  Inputs=3
  Mux4 : Mux  Inputs=5
  Rad2Deg : Gain  Gain=180/pi
  "Re-group " : Subsystem
  Zero : Gain  Gain=0
  Ref_JJVVAA : Outport
  RefEnd : Outport  Port=2
  Ref_JVAJVA : Outport  Port=3
  wires:
  Zero/1 -> Mux4/5, Mux4/3
  Mux6/1 -> Zero/1, Mux4/4
  Mux5/1 -> Mux4/2
  "Re-group "/1(JVAJVA) -> Rad2Deg/1
  Mux3/1 -> "Re-group "/1(JJVVAA), Ref_JJVVAA/1
  Derivative/1 -> Mux3/3
  Jacobian/1(Omega) -> Derivative/1, Mux3/2
  Mux1/1 -> Jacobian/2(EndVel)
  Derivative3/1 -> Mux6/3
  Drivative2/1 -> Mux6/2
  Derivative1/1 -> Mux6/1
  Mux4/1 -> RefEnd/1
  Inverse Kinematic/1(Theta) -> Mux3/1, Jacobian/1(Theta)
  Mux2/1 -> Mux4/1, Inverse Kinematic/1(EndPos)
  Integrator2/1 -> Mux2/3
  EndVelocity/3(EndVz) -> Mux5/3, Derivative3/1, Mux1/3, Integrator2/1
  EndVelocity/2(EndVy) -> Mux5/2, Drivative2/1, Mux1/2, Integrator1/1
  EndVelocity/1(EndVx) -> Mux5/1, Derivative1/1, Mux1/1, Integrator/1
  Integrator1/1 -> Mux2/2
  Integrator/1 -> Mux2/1
  Rad2Deg/1 -> Ref_JVAJVA/1

== system EulerPIDJoint_Copy/Controller/PID Controller/PID Controller ==
  Ref : Inport
  Enc : Inport  Port=2
  Chech Axis Error Flag : Logic  Inputs=6  AllPortsSameDT=off  OutDataTypeStr=boolean
  Controller Axis 1 : Subsystem  mask{RobotAxis=RobotAxis(1), Ts=Ts}
      mask prompts: RobotAxis "Robot Axis Controller Parameter"; Ts "Sample Time"
      mask init:
      | %% Source and Control Loop Selection
      | iPosCtl=RobotAxis.PosSourceSelect;
      | iVelCtl=RobotAxis.VelSourceSelect;
      | iCurrentCtl=RobotAxis.CurrentSourceSelect;
      | AxisNO=RobotAxis.AxisNO;
      | 
      | %% Controller Parameter
      | PLKp=RobotAxis.PLKp; % Kp for position loop
      | PLLimit=RobotAxis.PLLimit; 
      | 
      | VLKp = RobotAxis.VLKp; % Kp for velocity loop
      | VLKi = RobotAxis.VLKi;
      | VLLimit = RobotAxis.VLLimit;
      | 
      | Current2Volt=RobotAxis.Current2Volt;
      | 
      | %% Protection
      | VelErrorCheckLimit=RobotAxis.VelErrorCheckLimit;
  Controller Axis 2 : Subsystem  mask{RobotAxis=RobotAxis(2), Ts=Ts}
      mask prompts: RobotAxis "Robot Axis Controller Parameter"; Ts "Sample Time"
      mask init: same as EulerPIDJoint_Copy/Controller/PID Controller/PID Controller/Controller Axis 1
  Controller Axis 3 : Subsystem  mask{RobotAxis=RobotAxis(3), Ts=Ts}
      mask prompts: RobotAxis "Robot Axis Controller Parameter"; Ts "Sample Time"
      mask init: same as EulerPIDJoint_Copy/Controller/PID Controller/PID Controller/Controller Axis 1
  Controller Axis 4 : Subsystem  mask{RobotAxis=RobotAxis(4), Ts=Ts}
      mask prompts: RobotAxis "Robot Axis Controller Parameter"; Ts "Sample Time"
      mask init: same as EulerPIDJoint_Copy/Controller/PID Controller/PID Controller/Controller Axis 1
  Controller Axis 5 : Subsystem  mask{RobotAxis=RobotAxis(5), Ts=Ts}
      mask prompts: RobotAxis "Robot Axis Controller Parameter"; Ts "Sample Time"
      mask init: same as EulerPIDJoint_Copy/Controller/PID Controller/PID Controller/Controller Axis 1
  Controller Axis 6 : Subsystem  mask{RobotAxis=RobotAxis(6), Ts=Ts}
      mask prompts: RobotAxis "Robot Axis Controller Parameter"; Ts "Sample Time"
      mask init: same as EulerPIDJoint_Copy/Controller/PID Controller/PID Controller/Controller Axis 1
  Current2Volt : Gain  Gain=Rad2Line  SampleTime=Ts
  Current2Volt1 : Gain  Gain=Rad2Line  SampleTime=Ts
  Current2Volt2 : Gain  Gain=V2T
  Demux : Demux  Outputs=3
  Demux1 : Demux  Outputs=3
  Flag : Scope
      settings: TimeRange=12  YMin=-9  YMax=9
  Integer Delay : simulink/Discrete/Integer Delay  NumDelays=1  vinit=[a1;a2;a3;a4;a5;a6;0;0;0;0;0;0;0;0;0;0;0;0]/180*pi  samptime=Ts
  Mux : Mux  Inputs=6
  Source Model : Subsystem
  Terminator{,1..3} (4 alike) : Terminator
  Voltage : Scope
      settings: TimeRange=12  YMin=-9  YMax=9
  Feedback : Outport
  ErrorFlag : Outport  Port=2
  wires:
  Controller Axis 1/1(CurrentVolt) -> Mux/1  "Volt Axis1"
  Controller Axis 2/1(CurrentVolt) -> Mux/2  "Volt Axis2"
  Controller Axis 3/1(CurrentVolt) -> Mux/3  "Volt Axis3"
  Controller Axis 4/1(CurrentVolt) -> Mux/4  "Volt Axis4"
  Controller Axis 5/1(CurrentVolt) -> Mux/5  "Volt Axis5"
  Controller Axis 6/1(CurrentVolt) -> Mux/6  "Volt Axis6"
  Mux/1 -> Voltage/1, Current2Volt2/1
  Controller Axis 1/2(Axis Error Flag) -> Chech Axis Error Flag/1  "Error Axis1"
  Controller Axis 2/2(Axis Error Flag) -> Chech Axis Error Flag/2  "Error Axis2"
  Controller Axis 3/2(Axis Error Flag) -> Chech Axis Error Flag/3  "Error Axis3"
  Controller Axis 4/2(Axis Error Flag) -> Chech Axis Error Flag/4  "Error Axis4"
  Controller Axis 5/2(Axis Error Flag) -> Chech Axis Error Flag/5  "Error Axis5"
  Controller Axis 6/2(Axis Error Flag) -> Chech Axis Error Flag/6  "Error Axis6"
  Chech Axis Error Flag/1 -> ErrorFlag/1, Flag/1
  Current2Volt/1 -> Controller Axis 6/1(Prof), Controller Axis 5/1(Prof), Controller Axis 4/1(Prof), Controller Axis 3/1(Prof), Controller Axis 2/1(Prof), Controller Axis 1/1(Prof)
  Current2Volt1/1 -> Controller Axis 6/2(Enc), Controller Axis 5/2(Enc), Controller Axis 4/2(Enc), Controller Axis 3/2(Enc), Controller Axis 1/2(Enc), Controller Axis 2/2(Enc)
  Current2Volt2/1 -> Feedback/1
  Ref/1 -> Demux/1
  Demux/1 -> Current2Volt/1
  Demux/2 -> Terminator/1
  Demux/3 -> Terminator1/1
  Demux1/1 -> Current2Volt1/1
  Demux1/2 -> Terminator2/1
  Demux1/3 -> Terminator3/1
  Enc/1 -> Integer Delay/1
  Integer Delay/1 -> Demux1/1

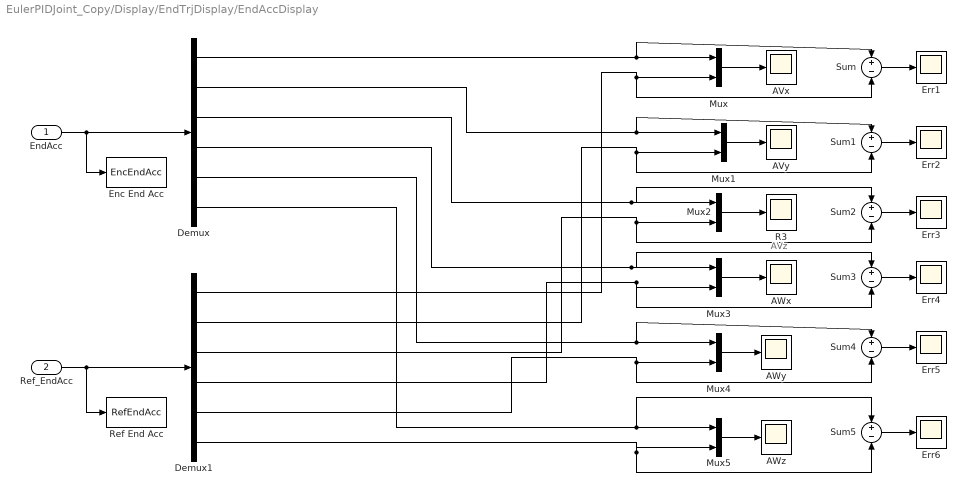
== system EulerPIDJoint_Copy/Display/EndTrjDisplay/EndAccDisplay ==
  note: AVz
  EndAcc : Inport
  Ref_EndAcc : Inport  Port=2
  AVx : Scope
      settings: TimeRange=10  YMin=-3e-017  YMax=4e-017
  "AVy " : Scope
  AWx : Scope
      settings: SaveName=ScopeData3
  AWy : Scope
      settings: TimeRange=10  YMin=-4.18  YMax=-4.04  SaveName=ScopeData4
  AWz : Scope
      settings: TimeRange=10  YMin=-1.6e-006  YMax=4e-007  SaveName=ScopeData5
  Demux : Demux  Outputs=6
  Demux1 : Demux  Outputs=6
  Enc End Acc : ToWorkspace  VariableName=EncEndAcc  SampleTime=-1  SaveFormat=Structure
  Err{1..6} (6 alike) : Scope
      Err1 settings: SaveName=ScopeData6
      Err2 settings: SaveName=ScopeData7
      Err3 settings: SaveName=ScopeData8
      Err4 settings: SaveName=ScopeData9
      Err5 settings: TimeRange=3  YMin=-2.5  YMax=1  SaveName=ScopeData10
      Err6 settings: SaveName=ScopeData11
  Mux{,1..5} (6 alike) : Mux  Inputs=2
  R3 : Scope
      settings: SaveName=ScopeData2
  Ref End Acc : ToWorkspace  VariableName=RefEndAcc  SampleTime=-1  SaveFormat=Structure
  Sum{,1..5} (6 alike) : Sum  Inputs=+|-
  wires:
  Mux5/1 -> AWz/1
  Mux4/1 -> AWy/1
  Mux3/1 -> AWx/1
  Mux2/1 -> R3/1
  Mux1/1 -> "AVy "/1
  Mux/1 -> AVx/1
  Sum/1 -> Err1/1
  Sum1/1 -> Err2/1
  Sum2/1 -> Err3/1
  Sum3/1 -> Err4/1
  Sum4/1 -> Err5/1
  Sum5/1 -> Err6/1
  EndAcc/1 -> Demux/1, Enc End Acc/1
  Ref_EndAcc/1 -> Demux1/1, Ref End Acc/1
  Demux/1 -> Mux/1, Sum/1
  Demux1/1 -> Mux/2, Sum/2
  Demux/2 -> Mux1/1, Sum1/1
  Demux/3 -> Mux2/1, Sum2/1
  Demux/4 -> Mux3/1, Sum3/1
  Demux/5 -> Mux4/1, Sum4/1
  Demux/6 -> Mux5/1, Sum5/1
  Demux1/2 -> Mux1/2, Sum1/2
  Demux1/3 -> Mux2/2, Sum2/2
  Demux1/4 -> Mux3/2, Sum3/2
  Demux1/5 -> Mux4/2, Sum4/2
  Demux1/6 -> Mux5/2, Sum5/2

== system EulerPIDJoint_Copy/Display/EndTrjDisplay/EndPosDisplay ==
  EndPos : Inport
  Ref_EndPos : Inport  Port=2
  Demux : Demux  Outputs=3
  Demux1 : Demux  Outputs=3
  "Encoder " : ToWorkspace  VariableName=EncEndPos  SampleTime=-1  SaveFormat=Structure
  Err1 : Scope
      settings: SaveName=ScopeData6
  Err2 : Scope
      settings: SaveName=ScopeData7
  Err3 : Scope
      settings: SaveName=ScopeData8
  Mux : Mux  Inputs=2
  Mux1 : Mux  Inputs=2
  Mux2 : Mux  Inputs=2
  "Ref " : ToWorkspace  VariableName=RefEndPos  SampleTime=-1  SaveFormat=Structure
  Sum : Sum  Inputs=+|-
  Sum1 : Sum  Inputs=+|-
  Sum2 : Sum  Inputs=+|-
  X : Scope
      settings: TimeRange=10  YMin=-3e-017  YMax=4e-017
  "Y " : Scope
      settings: YMin=-149  YMax=-136
  Z : Scope
      settings: SaveName=ScopeData2
  wires:
  Ref_EndPos/1 -> "Ref "/1, Demux1/1
  EndPos/1 -> "Encoder "/1, Demux/1
  Sum2/1 -> Err3/1
  Sum1/1 -> Err2/1
  Sum/1 -> Err1/1
  Demux/1 -> Sum/1, Mux/1
  Demux1/1 -> Sum/2, Mux/2
  Demux/2 -> Sum1/1, Mux1/1
  Demux1/2 -> Sum1/2, Mux1/2
  Demux/3 -> Sum2/1, Mux2/1
  Demux1/3 -> Sum2/2, Mux2/2
  Mux/1 -> X/1
  Mux1/1 -> "Y "/1
  Mux2/1 -> Z/1

== system EulerPIDJoint_Copy/Display/EndTrjDisplay/EndVelDisplay ==
  note: Vz
  EndVel : Inport
  Ref_EndVel : Inport  Port=2
  Demux : Demux  Outputs=6
  Demux1 : Demux  Outputs=6
  Enc End Vel : ToWorkspace  VariableName=EncEndVel  SampleTime=-1  SaveFormat=Structure
  Err{1..6} (6 alike) : Scope
      Err1 settings: SaveName=ScopeData6
      Err2 settings: SaveName=ScopeData7
      Err3 settings: SaveName=ScopeData8
      Err4 settings: SaveName=ScopeData9
      Err5 settings: TimeRange=3  YMin=-2.5  YMax=1  SaveName=ScopeData10
      Err6 settings: SaveName=ScopeData11
  Mux{,1..5} (6 alike) : Mux  Inputs=2
  R3 : Scope
      settings: SaveName=ScopeData2
  Ref End Vel : ToWorkspace  VariableName=RefEndVel  SampleTime=-1  SaveFormat=Structure
  Sum{,1..5} (6 alike) : Sum  Inputs=+|-
  Vx : Scope
      settings: TimeRange=10  YMin=-3e-017  YMax=4e-017
  "Vy " : Scope
      settings: TimeRange=8
  Wx : Scope
      settings: SaveName=ScopeData3
  Wy : Scope
      settings: TimeRange=10  YMin=-4.18  YMax=-4.04  SaveName=ScopeData4
  Wz : Scope
      settings: TimeRange=10  YMin=-1.6e-006  YMax=4e-007  SaveName=ScopeData5
  wires:
  Demux1/6 -> Sum5/2, Mux5/2
  Demux1/5 -> Sum4/2, Mux4/2
  Demux1/4 -> Sum3/2, Mux3/2
  Demux1/3 -> Sum2/2, Mux2/2
  Demux1/2 -> Sum1/2, Mux1/2
  Demux/6 -> Sum5/1, Mux5/1
  Demux/5 -> Sum4/1, Mux4/1
  Demux/4 -> Sum3/1, Mux3/1
  Demux/3 -> Sum2/1, Mux2/1
  Demux/2 -> Sum1/1, Mux1/1
  Demux1/1 -> Sum/2, Mux/2
  Demux/1 -> Sum/1, Mux/1
  Ref_EndVel/1 -> Ref End Vel/1, Demux1/1
  EndVel/1 -> Enc End Vel/1, Demux/1
  Sum5/1 -> Err6/1
  Sum4/1 -> Err5/1
  Sum3/1 -> Err4/1
  Sum2/1 -> Err3/1
  Sum1/1 -> Err2/1
  Sum/1 -> Err1/1
  Mux/1 -> Vx/1
  Mux1/1 -> "Vy "/1
  Mux2/1 -> R3/1
  Mux3/1 -> Wx/1
  Mux4/1 -> Wy/1
  Mux5/1 -> Wz/1

== system EulerPIDJoint_Copy/Display/GeneralAccDisplay/Jnt1 ==
  Enc : Inport
  Ref : Inport  Port=2
  Demux1 : Demux  Outputs=2
  Demux3 : Demux  Outputs=6
  Display : Subsystem
  Mux : Mux  Inputs=3
  Mux1 : Mux  Inputs=3
  Mux2 : Mux  Inputs=2
  Mux3 : Mux  Inputs=2
  Sign{1..6} (6 alike) : Gain
  wires:
  Mux3/1 -> Display/2(Ref_GeneralAcc1)
  Mux2/1 -> Display/1(GeneralAcc1)
  Sign6/1 -> Mux1/3
  Sign5/1 -> Mux1/2
  Sign4/1 -> Mux1/1
  Sign3/1 -> Mux/3
  Sign2/1 -> Mux/2
  Sign1/1 -> Mux/1
  Demux3/6 -> Sign6/1
  Demux3/5 -> Sign5/1
  Demux3/4 -> Sign4/1
  Demux3/3 -> Sign3/1
  Demux3/2 -> Sign2/1
  Demux3/1 -> Sign1/1
  Mux1/1 -> Mux3/2
  Mux/1 -> Mux3/1
  Ref/1 -> Demux3/1
  Enc/1 -> Demux1/1
  Demux1/1 -> Mux2/1
  Demux1/2 -> Mux2/2

== system EulerPIDJoint_Copy/Display/GeneralAccDisplay/Jnt2 ==
  Enc : Inport
  Ref : Inport  Port=2
  Demux1 : Demux  Outputs=2
  Demux3 : Demux  Outputs=6
  Display : Subsystem
  Mux : Mux  Inputs=3
  Mux1 : Mux  Inputs=3
  Mux2 : Mux  Inputs=2
  Mux3 : Mux  Inputs=2
  Sign{1..2,4..5} (4 alike) : Gain
  Sign3 : Gain  Gain=-1
  Sign6 : Gain  Gain=-1
  wires:
  Sign5/1 -> Mux1/3
  Sign6/1 -> Mux1/2
  Sign2/1 -> Mux/3
  Sign3/1 -> Mux/2
  Enc/1 -> Demux1/1
  Ref/1 -> Demux3/1
  Mux/1 -> Mux3/1
  Mux1/1 -> Mux3/2
  Demux3/1 -> Sign1/1
  Demux3/2 -> Sign2/1
  Demux3/3 -> Sign3/1
  Demux3/4 -> Sign4/1
  Demux3/5 -> Sign5/1
  Demux3/6 -> Sign6/1
  Sign1/1 -> Mux/1
  Sign4/1 -> Mux1/1
  Mux2/1 -> Display/1(GeneralAcc2)
  Mux3/1 -> Display/2(Ref_GeneralAcc2)
  Demux1/1 -> Mux2/1
  Demux1/2 -> Mux2/2

== system EulerPIDJoint_Copy/Display/GeneralAccDisplay/Jnt3 ==
  Enc : Inport
  Ref : Inport  Port=2
  Demux1 : Demux  Outputs=2
  Demux3 : Demux  Outputs=6
  Display : Subsystem
  Mux : Mux  Inputs=3
  Mux1 : Mux  Inputs=3
  Mux2 : Mux  Inputs=2
  Mux3 : Mux  Inputs=2
  Sign{1..6} (6 alike) : Gain
  wires:
  Sign5/1 -> Mux1/3
  Sign6/1 -> Mux1/1
  Sign4/1 -> Mux1/2
  Sign3/1 -> Mux/1
  Sign2/1 -> Mux/3
  Sign1/1 -> Mux/2
  Mux3/1 -> Display/2(Ref_GeneralAcc3)
  Mux2/1 -> Display/1(GeneralAcc3)
  Demux3/6 -> Sign6/1
  Demux3/5 -> Sign5/1
  Demux3/4 -> Sign4/1
  Demux3/3 -> Sign3/1
  Demux3/2 -> Sign2/1
  Demux3/1 -> Sign1/1
  Mux1/1 -> Mux3/2
  Mux/1 -> Mux3/1
  Ref/1 -> Demux3/1
  Enc/1 -> Demux1/1
  Demux1/1 -> Mux2/1
  Demux1/2 -> Mux2/2

== system EulerPIDJoint_Copy/Display/GeneralAccDisplay/Jnt4 ==
  Enc : Inport
  Ref : Inport  Port=2
  Demux1 : Demux  Outputs=2
  Demux3 : Demux  Outputs=6
  Display : Subsystem
  Mux : Mux  Inputs=3
  Mux1 : Mux  Inputs=3
  Mux2 : Mux  Inputs=2
  Mux3 : Mux  Inputs=2
  Sign{1,3..4,6} (4 alike) : Gain
  Sign2 : Gain  Gain=-1
  Sign5 : Gain  Gain=-1
  wires:
  Sign6/1 -> Mux1/1
  Sign4/1 -> Mux1/3
  Sign3/1 -> Mux/1
  Sign1/1 -> Mux/3
  Enc/1 -> Demux1/1
  Ref/1 -> Demux3/1
  Mux/1 -> Mux3/1
  Mux1/1 -> Mux3/2
  Demux3/1 -> Sign1/1
  Demux3/2 -> Sign2/1
  Demux3/3 -> Sign3/1
  Demux3/4 -> Sign4/1
  Demux3/5 -> Sign5/1
  Demux3/6 -> Sign6/1
  Sign2/1 -> Mux/2
  Sign5/1 -> Mux1/2
  Mux2/1 -> Display/1(GeneralAcc4)
  Mux3/1 -> Display/2(Ref_GeneralAcc4)
  Demux1/1 -> Mux2/1
  Demux1/2 -> Mux2/2

== system EulerPIDJoint_Copy/Display/GeneralAccDisplay/Jnt5 ==
  Enc : Inport
  Ref : Inport  Port=2
  Demux1 : Demux  Outputs=2
  Demux3 : Demux  Outputs=6
  Display : Subsystem
  Mux : Mux  Inputs=3
  Mux1 : Mux  Inputs=3
  Mux2 : Mux  Inputs=2
  Mux3 : Mux  Inputs=2
  Sign{1,3..4,6} (4 alike) : Gain  Gain=-1
  Sign2 : Gain
  Sign5 : Gain
  wires:
  Sign6/1 -> Mux1/1
  Sign5/1 -> Mux1/3
  Sign4/1 -> Mux1/2
  Sign3/1 -> Mux/1
  Sign2/1 -> Mux/3
  Sign1/1 -> Mux/2
  Mux3/1 -> Display/2(Ref_GeneralAcc5)
  Mux2/1 -> Display/1(GeneralAcc5)
  Demux3/6 -> Sign6/1
  Demux3/5 -> Sign5/1
  Demux3/4 -> Sign4/1
  Demux3/3 -> Sign3/1
  Demux3/2 -> Sign2/1
  Demux3/1 -> Sign1/1
  Mux1/1 -> Mux3/2
  Mux/1 -> Mux3/1
  Ref/1 -> Demux3/1
  Enc/1 -> Demux1/1
  Demux1/1 -> Mux2/1
  Demux1/2 -> Mux2/2

== system EulerPIDJoint_Copy/Display/GeneralAccDisplay/Jnt6 ==
  Enc : Inport
  Ref : Inport  Port=2
  Demux1 : Demux  Outputs=2
  Demux3 : Demux  Outputs=6
  Display : Subsystem
  Mux : Mux  Inputs=3
  Mux1 : Mux  Inputs=3
  Mux2 : Mux  Inputs=2
  Mux3 : Mux  Inputs=2
  Sign{1,3..4,6} (4 alike) : Gain
  Sign2 : Gain  Gain=-1
  Sign5 : Gain  Gain=-1
  wires:
  Sign4/1 -> Mux1/3
  Sign6/1 -> Mux1/1
  Sign3/1 -> Mux/1
  Sign1/1 -> Mux/3
  Enc/1 -> Demux1/1
  Ref/1 -> Demux3/1
  Mux/1 -> Mux3/1
  Mux1/1 -> Mux3/2
  Demux3/1 -> Sign1/1
  Demux3/2 -> Sign2/1
  Demux3/3 -> Sign3/1
  Demux3/4 -> Sign4/1
  Demux3/5 -> Sign5/1
  Demux3/6 -> Sign6/1
  Sign2/1 -> Mux/2
  Sign5/1 -> Mux1/2
  Mux2/1 -> Display/1(GeneralAcc6)
  Mux3/1 -> Display/2(Ref_GeneralAcc6)
  Demux1/1 -> Mux2/1
  Demux1/2 -> Mux2/2

== system EulerPIDJoint_Copy/Display/GeneralForceDisplay/Jnt1 ==
  Enc : Inport
  Ref : Inport  Port=2
  Demux1 : Demux  Outputs=2
  Demux3 : Demux  Outputs=6
  Display : Subsystem
  Mux : Mux  Inputs=3
  Mux1 : Mux  Inputs=3
  Mux2 : Mux  Inputs=2
  Mux3 : Mux  Inputs=2
  Sign{1..6} (6 alike) : Gain
  wires:
  Enc/1 -> Demux1/1
  Ref/1 -> Demux3/1
  Mux/1 -> Mux3/1
  Mux1/1 -> Mux3/2
  Demux3/1 -> Sign1/1
  Demux3/2 -> Sign2/1
  Demux3/3 -> Sign3/1
  Demux3/4 -> Sign4/1
  Demux3/5 -> Sign5/1
  Demux3/6 -> Sign6/1
  Sign1/1 -> Mux/1
  Sign2/1 -> Mux/2
  Sign3/1 -> Mux/3
  Sign4/1 -> Mux1/1
  Sign5/1 -> Mux1/2
  Sign6/1 -> Mux1/3
  Mux2/1 -> Display/1(GeneralForce1)
  Mux3/1 -> Display/2(Ref_GeneralForce1)
  Demux1/1 -> Mux2/1
  Demux1/2 -> Mux2/2

== system EulerPIDJoint_Copy/Display/GeneralForceDisplay/Jnt2 ==
  Enc : Inport
  Ref : Inport  Port=2
  Demux1 : Demux  Outputs=2
  Demux3 : Demux  Outputs=6
  Display : Subsystem
  Mux : Mux  Inputs=3
  Mux1 : Mux  Inputs=3
  Mux2 : Mux  Inputs=2
  Mux3 : Mux  Inputs=2
  Sign{1..2,4..5} (4 alike) : Gain
  Sign3 : Gain  Gain=-1
  Sign6 : Gain  Gain=-1
  wires:
  Mux3/1 -> Display/2(Ref_GeneralForce2)
  Mux2/1 -> Display/1(GeneralForce2)
  Sign4/1 -> Mux1/1
  Sign1/1 -> Mux/1
  Demux3/6 -> Sign6/1
  Demux3/5 -> Sign5/1
  Demux3/4 -> Sign4/1
  Demux3/3 -> Sign3/1
  Demux3/2 -> Sign2/1
  Demux3/1 -> Sign1/1
  Mux1/1 -> Mux3/2
  Mux/1 -> Mux3/1
  Ref/1 -> Demux3/1
  Enc/1 -> Demux1/1
  Sign3/1 -> Mux/2
  Sign2/1 -> Mux/3
  Sign6/1 -> Mux1/2
  Sign5/1 -> Mux1/3
  Demux1/1 -> Mux2/1
  Demux1/2 -> Mux2/2

== system EulerPIDJoint_Copy/Display/GeneralForceDisplay/Jnt3 ==
  Enc : Inport
  Ref : Inport  Port=2
  Demux1 : Demux  Outputs=2
  Demux3 : Demux  Outputs=6
  Display : Subsystem
  Mux : Mux  Inputs=3
  Mux1 : Mux  Inputs=3
  Mux2 : Mux  Inputs=2
  Mux3 : Mux  Inputs=2
  Sign{1..6} (6 alike) : Gain
  wires:
  Enc/1 -> Demux1/1
  Ref/1 -> Demux3/1
  Mux/1 -> Mux3/1
  Mux1/1 -> Mux3/2
  Demux3/1 -> Sign1/1
  Demux3/2 -> Sign2/1
  Demux3/3 -> Sign3/1
  Demux3/4 -> Sign4/1
  Demux3/5 -> Sign5/1
  Demux3/6 -> Sign6/1
  Mux2/1 -> Display/1(GeneralForce3)
  Mux3/1 -> Display/2(Ref_GeneralForce3)
  Sign1/1 -> Mux/2
  Sign2/1 -> Mux/3
  Sign3/1 -> Mux/1
  Sign4/1 -> Mux1/2
  Sign6/1 -> Mux1/1
  Sign5/1 -> Mux1/3
  Demux1/1 -> Mux2/1
  Demux1/2 -> Mux2/2
